simulink model "OAC_LA_Ass1_Task1_simu_R2017b"  (R2017b)
settings: Solver=VariableStepAuto  StartTime=0.0  StopTime=10.0  RelTol=1e-3
undefined symbols (not defined in the file): g, l, omega_0, phi_0
settings Model: Creator=miko2  LastModifiedBy=miko2

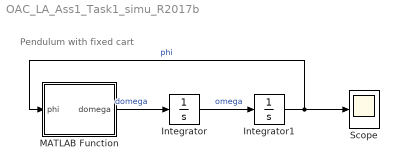
== system OAC_LA_Ass1_Task1_simu_R2017b ==
  note: Pendulum with fixed cart
  Integrator : Integrator  InitialCondition=omega_0
  Integrator1 : Integrator  InitialCondition=phi_0
  MATLAB Function : MATLAB Function  TreatAsAtomicUnit=on
  Scope : Scope
  wires:
  MATLAB Function/1(domega) -> Integrator/1  "domega"
  Integrator/1 -> Integrator1/1  "omega"
  Integrator1/1 -> Scope/1, MATLAB Function/1(phi)  "phi"

== matlab function OAC_LA_Ass1_Task1_simu_R2017b/MATLAB Function ==
  data: phi input size=3; domega output; g parameter; l parameter
function domega = fcn(phi,g, l)
    
    domega = g./ l .* sin(phi);
    
end
